simulink model "Inverse_model"  (R2021a)
settings: Solver=VariableStepAuto  StartTime=0.0  StopTime=1400  RelTol=1e-3
values from neighbouring files (symbols this model uses):
  B = 0.029    [project.m]
  J = 0.1    [project.m]
  ke = 0.6    [project.m]
  kt = 0.6    [project.m]
  La = 1e-3    (= 0.001)    [project.m]
  Ra = 1    [project.m]
libraries: pid_lib x6
settings Model: SimulationMode=rapid-accelerator  Creator=User  LastModifiedBy=User

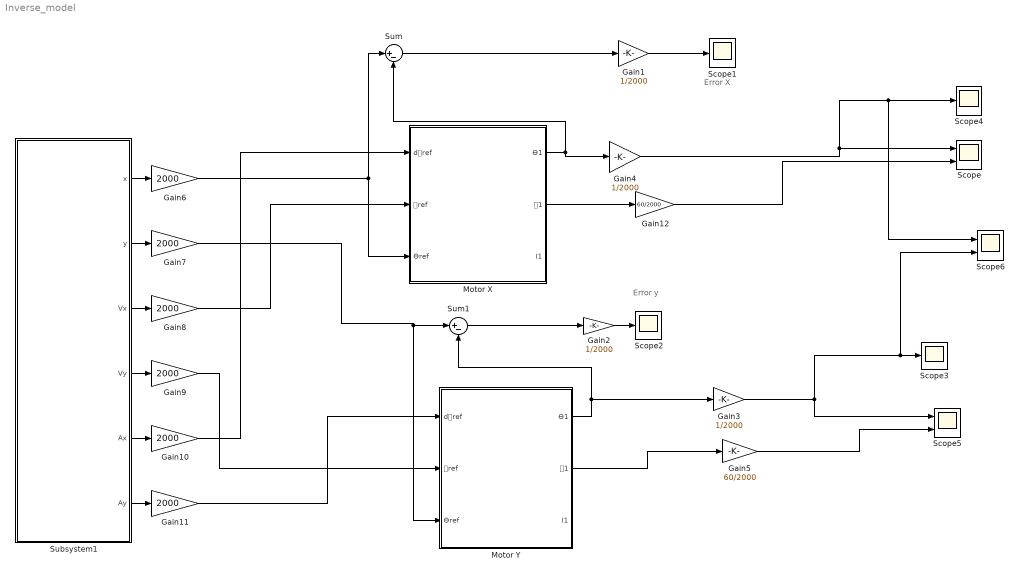
== system Inverse_model ==
  note: Error y
  note: Error X
  Gain{1..4} (4 alike) : Gain  Gain=1/2000
  Gain{6..11} (6 alike) : Gain  Gain=2000
  Gain12 : Gain  Gain=60/2000
  Gain5 : Gain  Gain=60/2000
  Motor X : Subsystem
  Motor Y : Subsystem
  Scope : Scope  NumInputPorts=2
  Scope{1..4} (4 alike) : Scope
  Scope5 : Scope  NumInputPorts=2
  Scope6 : Scope  NumInputPorts=2
  Subsystem1 : Subsystem
  Sum : Sum  Inputs=|+-
  Sum1 : Sum  Inputs=|+-
  wires:
  Subsystem1/1(x) -> Gain6/1
  Subsystem1/3(Vx) -> Gain8/1
  Subsystem1/5(Ax) -> Gain10/1
  Subsystem1/2(y) -> Gain7/1
  Subsystem1/4(Vy) -> Gain9/1
  Subsystem1/6(Ay) -> Gain11/1
  Sum1/1 -> Gain2/1
  Gain2/1 -> Scope2/1
  Gain3/1 -> Scope5/1, Scope6/2, Scope3/1
  Motor X/2(Ꞷ1) -> Gain12/1
  Gain6/1 -> Motor X/3(Ѳref), Sum/1
  Gain7/1 -> Sum1/1, Motor Y/3(Ѳref)
  Gain8/1 -> Motor X/2(Ꞷref)
  Gain10/1 -> Motor X/1(dꞶref)
  Gain9/1 -> Motor Y/2(Ꞷref)
  Gain11/1 -> Motor Y/1(dꞶref)
  Gain5/1 -> Scope5/2
  Motor X/1(Ѳ1) -> Gain4/1, Sum/2
  Gain4/1 -> Scope/1, Scope6/1, Scope4/1
  Sum/1 -> Gain1/1
  Gain1/1 -> Scope1/1
  Gain12/1 -> Scope/2
  Motor Y/1(Ѳ1) -> Gain3/1, Sum1/2
  Motor Y/2(Ꞷ1) -> Gain5/1

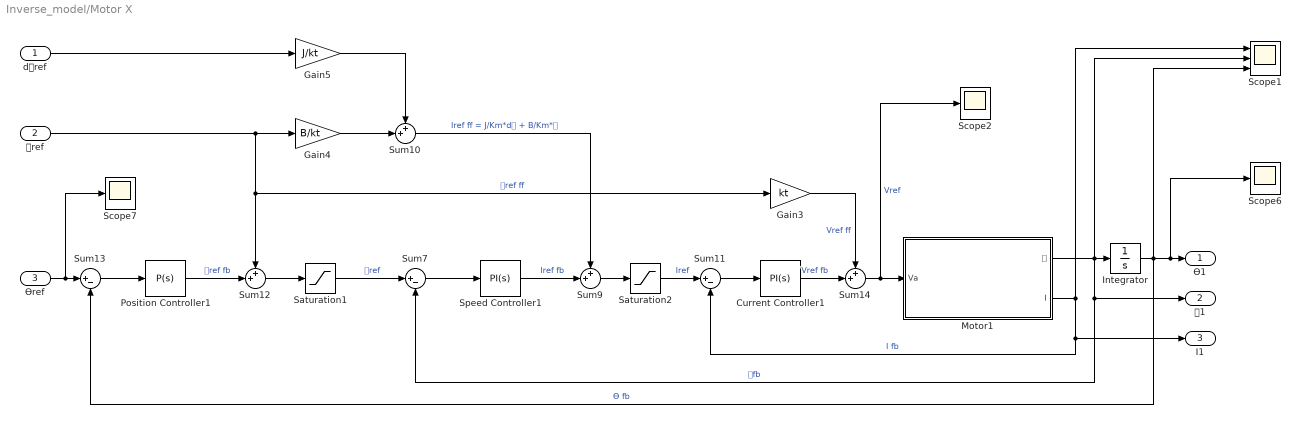
== system Inverse_model/Motor X ==
  dꞶref : Inport
  Ꞷref : Inport  Port=2
  Ѳref : Inport  Port=3
  Current Controller1 : pid_lib/PID Controller  Controller=PI  Form=Parallel  TimeDomain=Continuous-time  UseExternalTs=off  SampleTime=-1  IntegratorMethod=Forward Euler  FilterMethod=Forward Euler  ControllerParametersSource=internal  P=1000*La  I=1000*Ra  D=0  UseFilter=on  N=100  TunerSelectOption=Frequency Response Based  InitialConditionSource=internal  InitialConditionForIntegrator=0  InitialConditionForFilter=0  DifferentiatorICPrevScaledInput=0  ExternalReset=none  TrackingMode=off  Kt=1  LimitOutput=off  SatLimitsSource=internal  UpperSaturationLimit=inf  LowerSaturationLimit=-inf  LinearizeAsGain=on  AntiWindupMode=none  Kb=1  POutMin=[]  POutMax=[]  IOutMin=[]  IOutMax=[]  DOutMin=[]  DOutMax=[]  NOutMin=[]  NOutMax=[]  SumOutMin=[]  SumOutMax=[]  SaturationOutMin=[]  SaturationOutMax=[]  PParamMin=[]  PParamMax=[]  IParamMin=[]  IParamMax=[]  DParamMin=[]  DParamMax=[]  NParamMin=[]  NParamMax=[]  KbParamMin=[]  KbParamMax=[]  KtParamMin=[]  KtParamMax=[]  KbOutMin=[]  KbOutMax=[]  KtOutMin=[]  KtOutMax=[]  IntegratorOutMin=[]  IntegratorOutMax=[]  FilterOutMin=[]  FilterOutMax=[]  SumI1OutMin=[]  SumI1OutMax=[]  SumI2OutMin=[]  SumI2OutMax=[]  SumI3OutMin=[]  SumI3OutMax=[]  SumI4OutMin=[]  SumI4OutMax=[]  SumDOutMin=[]  SumDOutMax=[]  DifferentiatorOutMin=[]  DifferentiatorOutMax=[]  FilterDiffOutCoefMin=[]  FilterDiffOutCoefMax=[]  ReciprocalOutMin=[]  ReciprocalOutMax=[]  SumDenOutMin=[]  SumDenOutMax=[]  SumNumOutMin=[]  SumNumOutMax=[]  DivideOutMin=[]  DivideOutMax=[]  UdiffTsProdOutMin=[]  UdiffTsProdOutMax=[]  NTsProdOutMin=[]  NTsProdOutMax=[]  UintegralTsProdOutMin=[]  UintegralTsProdOutMax=[]  UngainTsProdOutMin=[]  UngainTsProdOutMax=[]  IntegratorContinuousStateAttributes=''  IntegratorStateMustResolveToSignalObject=off  IntegratorRTWStateStorageClass=Auto  FilterContinuousStateAttributes=''  FilterStateMustResolveToSignalObject=off  FilterRTWStateStorageClass=Auto  ParallelPVariant=InternalParameters  IdealPVariant=Disabled  IVariant=InternalParameters  DVariant=Disabled  IntegratorVariant=Continuous  SatVariant=Disabled  AWVariant=Passthrough  PCopyVariant=Disabled  TRVariant=Disabled  FdbkBlocksVariant=Forward  IdealPFdbkVariant=Disabled  SatFdbkVariant=Disabled  DerivativeFilterVariant=Disabled  NVariant=Disabled  NCopyVariant=Disabled_SignalSpec  FilterICVariant=Disabled  IntegratorICVariant=InternalICs  ExternalResetVariant=Disabled  TRSumVariant=Passthrough  SumFdbkVariant=Disabled  SumVariant=Sum_PI  TsampFilterVariant=InternalTs  TsampNgainVariant=Passthrough  TsampIntegralVariant=Passthrough  ExternalSaturationOutDataTypeStr=Inherit: Same as second input
  Gain3 : Gain  Gain=kt
  Gain4 : Gain  Gain=B/kt
  Gain5 : Gain  Gain=J/kt
  Integrator : Integrator  InitialCondition=6000
  Motor1 : Subsystem
  Position Controller1 : pid_lib/PID Controller  Controller=P  Form=Parallel  TimeDomain=Continuous-time  UseExternalTs=off  SampleTime=-1  IntegratorMethod=Forward Euler  FilterMethod=Forward Euler  ControllerParametersSource=internal  P=10  I=1  D=0  UseFilter=on  N=100  TunerSelectOption=Frequency Response Based  InitialConditionSource=internal  InitialConditionForIntegrator=0  InitialConditionForFilter=0  DifferentiatorICPrevScaledInput=0  ExternalReset=none  TrackingMode=off  Kt=1  LimitOutput=off  SatLimitsSource=internal  UpperSaturationLimit=inf  LowerSaturationLimit=-inf  LinearizeAsGain=on  AntiWindupMode=none  Kb=1  POutMin=[]  POutMax=[]  IOutMin=[]  IOutMax=[]  DOutMin=[]  DOutMax=[]  NOutMin=[]  NOutMax=[]  SumOutMin=[]  SumOutMax=[]  SaturationOutMin=[]  SaturationOutMax=[]  PParamMin=[]  PParamMax=[]  IParamMin=[]  IParamMax=[]  DParamMin=[]  DParamMax=[]  NParamMin=[]  NParamMax=[]  KbParamMin=[]  KbParamMax=[]  KtParamMin=[]  KtParamMax=[]  KbOutMin=[]  KbOutMax=[]  KtOutMin=[]  KtOutMax=[]  IntegratorOutMin=[]  IntegratorOutMax=[]  FilterOutMin=[]  FilterOutMax=[]  SumI1OutMin=[]  SumI1OutMax=[]  SumI2OutMin=[]  SumI2OutMax=[]  SumI3OutMin=[]  SumI3OutMax=[]  SumI4OutMin=[]  SumI4OutMax=[]  SumDOutMin=[]  SumDOutMax=[]  DifferentiatorOutMin=[]  DifferentiatorOutMax=[]  FilterDiffOutCoefMin=[]  FilterDiffOutCoefMax=[]  ReciprocalOutMin=[]  ReciprocalOutMax=[]  SumDenOutMin=[]  SumDenOutMax=[]  SumNumOutMin=[]  SumNumOutMax=[]  DivideOutMin=[]  DivideOutMax=[]  UdiffTsProdOutMin=[]  UdiffTsProdOutMax=[]  NTsProdOutMin=[]  NTsProdOutMax=[]  UintegralTsProdOutMin=[]  UintegralTsProdOutMax=[]  UngainTsProdOutMin=[]  UngainTsProdOutMax=[]  IntegratorContinuousStateAttributes=''  IntegratorStateMustResolveToSignalObject=off  IntegratorRTWStateStorageClass=Auto  FilterContinuousStateAttributes=''  FilterStateMustResolveToSignalObject=off  FilterRTWStateStorageClass=Auto  ParallelPVariant=InternalParameters  IdealPVariant=Disabled  IVariant=Disabled  DVariant=Disabled  IntegratorVariant=Disabled  SatVariant=Disabled  AWVariant=Disabled  PCopyVariant=Disabled  TRVariant=Disabled  FdbkBlocksVariant=Forward  IdealPFdbkVariant=Disabled  SatFdbkVariant=Disabled  DerivativeFilterVariant=Disabled  NVariant=Disabled  NCopyVariant=Disabled_SignalSpec  FilterICVariant=Disabled  IntegratorICVariant=Disabled  ExternalResetVariant=Disabled  TRSumVariant=Passthrough  SumFdbkVariant=Disabled  SumVariant=Passthrough_P  TsampFilterVariant=InternalTs  TsampNgainVariant=Passthrough  TsampIntegralVariant=Disabled_SignalSpec  ExternalSaturationOutDataTypeStr=Inherit: Same as second input
  Saturation1 : Saturate  UpperLimit=3000  LowerLimit=-3000
  Saturation2 : Saturate  UpperLimit=3000  LowerLimit=-3000
  Scope1 : Scope  NumInputPorts=3
  Scope2 : Scope
  Scope6 : Scope
  Scope7 : Scope
  Speed Controller1 : pid_lib/PID Controller  Controller=PI  Form=Parallel  TimeDomain=Continuous-time  UseExternalTs=off  SampleTime=-1  IntegratorMethod=Forward Euler  FilterMethod=Forward Euler  ControllerParametersSource=internal  P=344*J  I=344*B  D=2.5  UseFilter=on  N=100  TunerSelectOption=Transfer Function Based (PID Tuner App)  InitialConditionSource=internal  InitialConditionForIntegrator=0  InitialConditionForFilter=0  DifferentiatorICPrevScaledInput=0  ExternalReset=none  TrackingMode=off  Kt=1  LimitOutput=off  SatLimitsSource=internal  UpperSaturationLimit=inf  LowerSaturationLimit=-inf  LinearizeAsGain=on  AntiWindupMode=none  Kb=1  POutMin=[]  POutMax=[]  IOutMin=[]  IOutMax=[]  DOutMin=[]  DOutMax=[]  NOutMin=[]  NOutMax=[]  SumOutMin=[]  SumOutMax=[]  SaturationOutMin=[]  SaturationOutMax=[]  PParamMin=[]  PParamMax=[]  IParamMin=[]  IParamMax=[]  DParamMin=[]  DParamMax=[]  NParamMin=[]  NParamMax=[]  KbParamMin=[]  KbParamMax=[]  KtParamMin=[]  KtParamMax=[]  KbOutMin=[]  KbOutMax=[]  KtOutMin=[]  KtOutMax=[]  IntegratorOutMin=[]  IntegratorOutMax=[]  FilterOutMin=[]  FilterOutMax=[]  SumI1OutMin=[]  SumI1OutMax=[]  SumI2OutMin=[]  SumI2OutMax=[]  SumI3OutMin=[]  SumI3OutMax=[]  SumI4OutMin=[]  SumI4OutMax=[]  SumDOutMin=[]  SumDOutMax=[]  DifferentiatorOutMin=[]  DifferentiatorOutMax=[]  FilterDiffOutCoefMin=[]  FilterDiffOutCoefMax=[]  ReciprocalOutMin=[]  ReciprocalOutMax=[]  SumDenOutMin=[]  SumDenOutMax=[]  SumNumOutMin=[]  SumNumOutMax=[]  DivideOutMin=[]  DivideOutMax=[]  UdiffTsProdOutMin=[]  UdiffTsProdOutMax=[]  NTsProdOutMin=[]  NTsProdOutMax=[]  UintegralTsProdOutMin=[]  UintegralTsProdOutMax=[]  UngainTsProdOutMin=[]  UngainTsProdOutMax=[]  IntegratorContinuousStateAttributes=''  IntegratorStateMustResolveToSignalObject=off  IntegratorRTWStateStorageClass=Auto  FilterContinuousStateAttributes=''  FilterStateMustResolveToSignalObject=off  FilterRTWStateStorageClass=Auto  ParallelPVariant=InternalParameters  IdealPVariant=Disabled  IVariant=InternalParameters  DVariant=Disabled  IntegratorVariant=Continuous  SatVariant=Disabled  AWVariant=Passthrough  PCopyVariant=Disabled  TRVariant=Disabled  FdbkBlocksVariant=Forward  IdealPFdbkVariant=Disabled  SatFdbkVariant=Disabled  DerivativeFilterVariant=Disabled  NVariant=Disabled  NCopyVariant=Disabled_SignalSpec  FilterICVariant=Disabled  IntegratorICVariant=InternalICs  ExternalResetVariant=Disabled  TRSumVariant=Passthrough  SumFdbkVariant=Disabled  SumVariant=Sum_PI  TsampFilterVariant=InternalTs  TsampNgainVariant=Passthrough  TsampIntegralVariant=Passthrough  ExternalSaturationOutDataTypeStr=Inherit: Same as second input
  Sum{9..10,12,14} (4 alike) : Sum  Inputs=++|
  Sum11 : Sum  Inputs=|+-
  Sum13 : Sum  Inputs=|+-
  Sum7 : Sum  Inputs=|+-
  Ѳ1 : Outport  VectorParamsAs1DForOutWhenUnconnected=off
  Ꞷ1 : Outport  Port=2  VectorParamsAs1DForOutWhenUnconnected=off
  I1 : Outport  Port=3  VectorParamsAs1DForOutWhenUnconnected=off
  wires:
  Current Controller1/1 -> Sum14/2  "Vref fb"
  Sum10/1 -> Sum9/1  "Iref ff = J/Km*dꞶ + B/Km*Ꞷ"
  Gain3/1 -> Sum14/1  "Vref ff"
  Motor1/1(Ꞷ) -> Scope1/2, Integrator/1, Sum7/2, Ꞷ1/1  "Ꞷfb"
  Saturation2/1 -> Sum11/1  "Iref"
  Integrator/1 -> Scope1/3, Scope6/1, Ѳ1/1, Sum13/2  "Ѳ fb"
  Speed Controller1/1 -> Sum9/2  "Iref fb"
  Gain4/1 -> Sum10/2
  Position Controller1/1 -> Sum12/2  "Ꞷref fb"
  Ꞷref/1 -> Gain3/1, Sum12/1, Gain4/1  "Ꞷref ff"
  Motor1/2(I) -> Scope1/1, I1/1, Sum11/2  "I fb"
  dꞶref/1 -> Gain5/1
  Ѳref/1 -> Scope7/1, Sum13/1
  Sum12/1 -> Saturation1/1
  Gain5/1 -> Sum10/1
  Sum11/1 -> Current Controller1/1
  Sum7/1 -> Speed Controller1/1
  Sum14/1 -> Scope2/1, Motor1/1(Va)  "Vref"
  Sum9/1 -> Saturation2/1
  Sum13/1 -> Position Controller1/1
  Saturation1/1 -> Sum7/1  "Ꞷref"

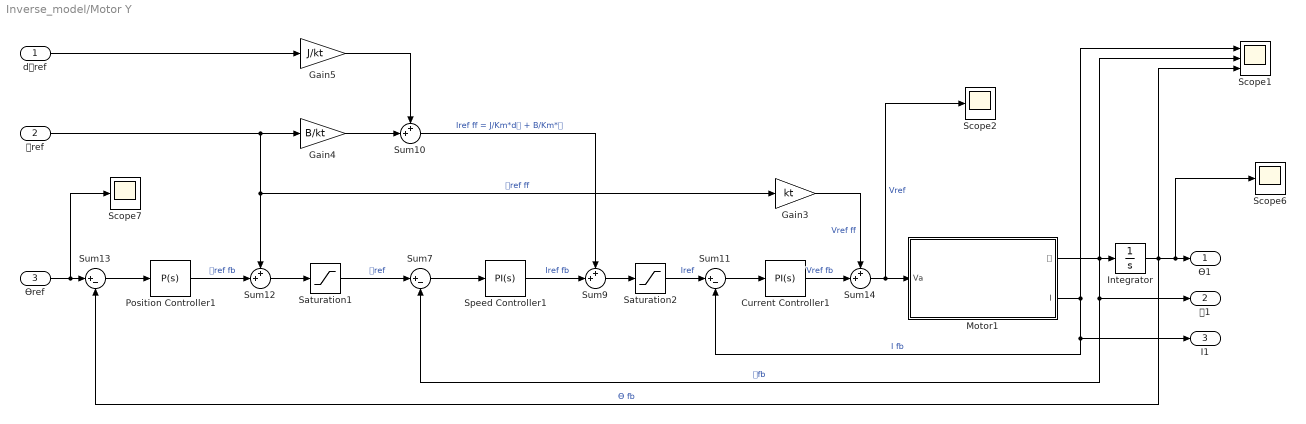
== system Inverse_model/Motor Y ==
  dꞶref : Inport
  Ꞷref : Inport  Port=2
  Ѳref : Inport  Port=3
  Current Controller1 : pid_lib/PID Controller  Controller=PI  Form=Parallel  TimeDomain=Continuous-time  UseExternalTs=off  SampleTime=-1  IntegratorMethod=Forward Euler  FilterMethod=Forward Euler  ControllerParametersSource=internal  P=1000*La  I=1000*Ra  D=0  UseFilter=on  N=100  TunerSelectOption=Frequency Response Based  InitialConditionSource=internal  InitialConditionForIntegrator=0  InitialConditionForFilter=0  DifferentiatorICPrevScaledInput=0  ExternalReset=none  TrackingMode=off  Kt=1  LimitOutput=off  SatLimitsSource=internal  UpperSaturationLimit=inf  LowerSaturationLimit=-inf  LinearizeAsGain=on  AntiWindupMode=none  Kb=1  POutMin=[]  POutMax=[]  IOutMin=[]  IOutMax=[]  DOutMin=[]  DOutMax=[]  NOutMin=[]  NOutMax=[]  SumOutMin=[]  SumOutMax=[]  SaturationOutMin=[]  SaturationOutMax=[]  PParamMin=[]  PParamMax=[]  IParamMin=[]  IParamMax=[]  DParamMin=[]  DParamMax=[]  NParamMin=[]  NParamMax=[]  KbParamMin=[]  KbParamMax=[]  KtParamMin=[]  KtParamMax=[]  KbOutMin=[]  KbOutMax=[]  KtOutMin=[]  KtOutMax=[]  IntegratorOutMin=[]  IntegratorOutMax=[]  FilterOutMin=[]  FilterOutMax=[]  SumI1OutMin=[]  SumI1OutMax=[]  SumI2OutMin=[]  SumI2OutMax=[]  SumI3OutMin=[]  SumI3OutMax=[]  SumI4OutMin=[]  SumI4OutMax=[]  SumDOutMin=[]  SumDOutMax=[]  DifferentiatorOutMin=[]  DifferentiatorOutMax=[]  FilterDiffOutCoefMin=[]  FilterDiffOutCoefMax=[]  ReciprocalOutMin=[]  ReciprocalOutMax=[]  SumDenOutMin=[]  SumDenOutMax=[]  SumNumOutMin=[]  SumNumOutMax=[]  DivideOutMin=[]  DivideOutMax=[]  UdiffTsProdOutMin=[]  UdiffTsProdOutMax=[]  NTsProdOutMin=[]  NTsProdOutMax=[]  UintegralTsProdOutMin=[]  UintegralTsProdOutMax=[]  UngainTsProdOutMin=[]  UngainTsProdOutMax=[]  IntegratorContinuousStateAttributes=''  IntegratorStateMustResolveToSignalObject=off  IntegratorRTWStateStorageClass=Auto  FilterContinuousStateAttributes=''  FilterStateMustResolveToSignalObject=off  FilterRTWStateStorageClass=Auto  ParallelPVariant=InternalParameters  IdealPVariant=Disabled  IVariant=InternalParameters  DVariant=Disabled  IntegratorVariant=Continuous  SatVariant=Disabled  AWVariant=Passthrough  PCopyVariant=Disabled  TRVariant=Disabled  FdbkBlocksVariant=Forward  IdealPFdbkVariant=Disabled  SatFdbkVariant=Disabled  DerivativeFilterVariant=Disabled  NVariant=Disabled  NCopyVariant=Disabled_SignalSpec  FilterICVariant=Disabled  IntegratorICVariant=InternalICs  ExternalResetVariant=Disabled  TRSumVariant=Passthrough  SumFdbkVariant=Disabled  SumVariant=Sum_PI  TsampFilterVariant=InternalTs  TsampNgainVariant=Passthrough  TsampIntegralVariant=Passthrough  ExternalSaturationOutDataTypeStr=Inherit: Same as second input
  Gain3 : Gain  Gain=kt
  Gain4 : Gain  Gain=B/kt
  Gain5 : Gain  Gain=J/kt
  Integrator : Integrator  InitialCondition=4000
  Motor1 : Subsystem
  Position Controller1 : pid_lib/PID Controller  Controller=P  Form=Parallel  TimeDomain=Continuous-time  UseExternalTs=off  SampleTime=-1  IntegratorMethod=Forward Euler  FilterMethod=Forward Euler  ControllerParametersSource=internal  P=10  I=1  D=0  UseFilter=on  N=100  TunerSelectOption=Frequency Response Based  InitialConditionSource=internal  InitialConditionForIntegrator=0  InitialConditionForFilter=0  DifferentiatorICPrevScaledInput=0  ExternalReset=none  TrackingMode=off  Kt=1  LimitOutput=off  SatLimitsSource=internal  UpperSaturationLimit=inf  LowerSaturationLimit=-inf  LinearizeAsGain=on  AntiWindupMode=none  Kb=1  POutMin=[]  POutMax=[]  IOutMin=[]  IOutMax=[]  DOutMin=[]  DOutMax=[]  NOutMin=[]  NOutMax=[]  SumOutMin=[]  SumOutMax=[]  SaturationOutMin=[]  SaturationOutMax=[]  PParamMin=[]  PParamMax=[]  IParamMin=[]  IParamMax=[]  DParamMin=[]  DParamMax=[]  NParamMin=[]  NParamMax=[]  KbParamMin=[]  KbParamMax=[]  KtParamMin=[]  KtParamMax=[]  KbOutMin=[]  KbOutMax=[]  KtOutMin=[]  KtOutMax=[]  IntegratorOutMin=[]  IntegratorOutMax=[]  FilterOutMin=[]  FilterOutMax=[]  SumI1OutMin=[]  SumI1OutMax=[]  SumI2OutMin=[]  SumI2OutMax=[]  SumI3OutMin=[]  SumI3OutMax=[]  SumI4OutMin=[]  SumI4OutMax=[]  SumDOutMin=[]  SumDOutMax=[]  DifferentiatorOutMin=[]  DifferentiatorOutMax=[]  FilterDiffOutCoefMin=[]  FilterDiffOutCoefMax=[]  ReciprocalOutMin=[]  ReciprocalOutMax=[]  SumDenOutMin=[]  SumDenOutMax=[]  SumNumOutMin=[]  SumNumOutMax=[]  DivideOutMin=[]  DivideOutMax=[]  UdiffTsProdOutMin=[]  UdiffTsProdOutMax=[]  NTsProdOutMin=[]  NTsProdOutMax=[]  UintegralTsProdOutMin=[]  UintegralTsProdOutMax=[]  UngainTsProdOutMin=[]  UngainTsProdOutMax=[]  IntegratorContinuousStateAttributes=''  IntegratorStateMustResolveToSignalObject=off  IntegratorRTWStateStorageClass=Auto  FilterContinuousStateAttributes=''  FilterStateMustResolveToSignalObject=off  FilterRTWStateStorageClass=Auto  ParallelPVariant=InternalParameters  IdealPVariant=Disabled  IVariant=Disabled  DVariant=Disabled  IntegratorVariant=Disabled  SatVariant=Disabled  AWVariant=Disabled  PCopyVariant=Disabled  TRVariant=Disabled  FdbkBlocksVariant=Forward  IdealPFdbkVariant=Disabled  SatFdbkVariant=Disabled  DerivativeFilterVariant=Disabled  NVariant=Disabled  NCopyVariant=Disabled_SignalSpec  FilterICVariant=Disabled  IntegratorICVariant=Disabled  ExternalResetVariant=Disabled  TRSumVariant=Passthrough  SumFdbkVariant=Disabled  SumVariant=Passthrough_P  TsampFilterVariant=InternalTs  TsampNgainVariant=Passthrough  TsampIntegralVariant=Disabled_SignalSpec  ExternalSaturationOutDataTypeStr=Inherit: Same as second input
  Saturation1 : Saturate  UpperLimit=3000  LowerLimit=-3000
  Saturation2 : Saturate  UpperLimit=3000  LowerLimit=-3000
  Scope1 : Scope  NumInputPorts=3
  Scope2 : Scope
  Scope6 : Scope
  Scope7 : Scope
  Speed Controller1 : pid_lib/PID Controller  Controller=PI  Form=Parallel  TimeDomain=Continuous-time  UseExternalTs=off  SampleTime=-1  IntegratorMethod=Forward Euler  FilterMethod=Forward Euler  ControllerParametersSource=internal  P=344*J  I=344*B  D=2.5  UseFilter=on  N=100  TunerSelectOption=Transfer Function Based (PID Tuner App)  InitialConditionSource=internal  InitialConditionForIntegrator=0  InitialConditionForFilter=0  DifferentiatorICPrevScaledInput=0  ExternalReset=none  TrackingMode=off  Kt=1  LimitOutput=off  SatLimitsSource=internal  UpperSaturationLimit=inf  LowerSaturationLimit=-inf  LinearizeAsGain=on  AntiWindupMode=none  Kb=1  POutMin=[]  POutMax=[]  IOutMin=[]  IOutMax=[]  DOutMin=[]  DOutMax=[]  NOutMin=[]  NOutMax=[]  SumOutMin=[]  SumOutMax=[]  SaturationOutMin=[]  SaturationOutMax=[]  PParamMin=[]  PParamMax=[]  IParamMin=[]  IParamMax=[]  DParamMin=[]  DParamMax=[]  NParamMin=[]  NParamMax=[]  KbParamMin=[]  KbParamMax=[]  KtParamMin=[]  KtParamMax=[]  KbOutMin=[]  KbOutMax=[]  KtOutMin=[]  KtOutMax=[]  IntegratorOutMin=[]  IntegratorOutMax=[]  FilterOutMin=[]  FilterOutMax=[]  SumI1OutMin=[]  SumI1OutMax=[]  SumI2OutMin=[]  SumI2OutMax=[]  SumI3OutMin=[]  SumI3OutMax=[]  SumI4OutMin=[]  SumI4OutMax=[]  SumDOutMin=[]  SumDOutMax=[]  DifferentiatorOutMin=[]  DifferentiatorOutMax=[]  FilterDiffOutCoefMin=[]  FilterDiffOutCoefMax=[]  ReciprocalOutMin=[]  ReciprocalOutMax=[]  SumDenOutMin=[]  SumDenOutMax=[]  SumNumOutMin=[]  SumNumOutMax=[]  DivideOutMin=[]  DivideOutMax=[]  UdiffTsProdOutMin=[]  UdiffTsProdOutMax=[]  NTsProdOutMin=[]  NTsProdOutMax=[]  UintegralTsProdOutMin=[]  UintegralTsProdOutMax=[]  UngainTsProdOutMin=[]  UngainTsProdOutMax=[]  IntegratorContinuousStateAttributes=''  IntegratorStateMustResolveToSignalObject=off  IntegratorRTWStateStorageClass=Auto  FilterContinuousStateAttributes=''  FilterStateMustResolveToSignalObject=off  FilterRTWStateStorageClass=Auto  ParallelPVariant=InternalParameters  IdealPVariant=Disabled  IVariant=InternalParameters  DVariant=Disabled  IntegratorVariant=Continuous  SatVariant=Disabled  AWVariant=Passthrough  PCopyVariant=Disabled  TRVariant=Disabled  FdbkBlocksVariant=Forward  IdealPFdbkVariant=Disabled  SatFdbkVariant=Disabled  DerivativeFilterVariant=Disabled  NVariant=Disabled  NCopyVariant=Disabled_SignalSpec  FilterICVariant=Disabled  IntegratorICVariant=InternalICs  ExternalResetVariant=Disabled  TRSumVariant=Passthrough  SumFdbkVariant=Disabled  SumVariant=Sum_PI  TsampFilterVariant=InternalTs  TsampNgainVariant=Passthrough  TsampIntegralVariant=Passthrough  ExternalSaturationOutDataTypeStr=Inherit: Same as second input
  Sum{9..10,12,14} (4 alike) : Sum  Inputs=++|
  Sum11 : Sum  Inputs=|+-
  Sum13 : Sum  Inputs=|+-
  Sum7 : Sum  Inputs=|+-
  Ѳ1 : Outport  VectorParamsAs1DForOutWhenUnconnected=off
  Ꞷ1 : Outport  Port=2  VectorParamsAs1DForOutWhenUnconnected=off
  I1 : Outport  Port=3  VectorParamsAs1DForOutWhenUnconnected=off
  wires:
  Saturation1/1 -> Sum7/1  "Ꞷref"
  Sum13/1 -> Position Controller1/1
  Sum11/1 -> Current Controller1/1
  Gain5/1 -> Sum10/1
  Sum12/1 -> Saturation1/1
  Gain4/1 -> Sum10/2
  Speed Controller1/1 -> Sum9/2  "Iref fb"
  Position Controller1/1 -> Sum12/2  "Ꞷref fb"
  Sum9/1 -> Saturation2/1
  Saturation2/1 -> Sum11/1  "Iref"
  Gain3/1 -> Sum14/1  "Vref ff"
  Motor1/1(Ꞷ) -> Scope1/2, Integrator/1, Sum7/2, Ꞷ1/1  "Ꞷfb"
  Sum14/1 -> Scope2/1, Motor1/1(Va)  "Vref"
  Current Controller1/1 -> Sum14/2  "Vref fb"
  Sum7/1 -> Speed Controller1/1
  Sum10/1 -> Sum9/1  "Iref ff = J/Km*dꞶ + B/Km*Ꞷ"
  Integrator/1 -> Scope1/3, Scope6/1, Ѳ1/1, Sum13/2  "Ѳ fb"
  Ꞷref/1 -> Gain3/1, Sum12/1, Gain4/1  "Ꞷref ff"
  dꞶref/1 -> Gain5/1
  Ѳref/1 -> Scope7/1, Sum13/1
  Motor1/2(I) -> Scope1/1, I1/1, Sum11/2  "I fb"

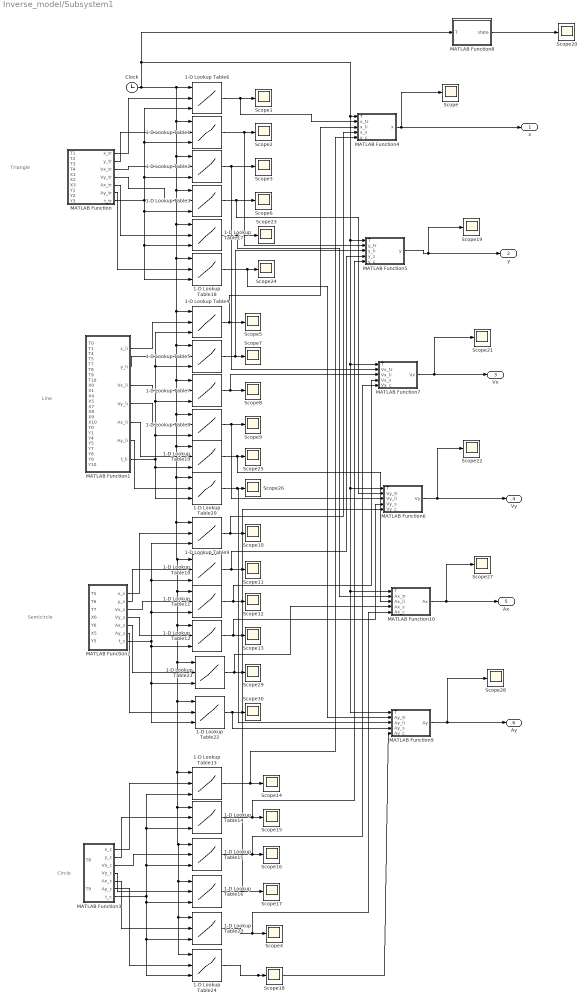
== system Inverse_model/Subsystem1 ==
  note: Circle
  note: Semicircle
  note: Line
  note: Triangle
  1-D Lookup Table{1..24} (24 alike) : Lookup_n-D  NumberOfTableDimensions=1  BreakpointsForDimension1Source=Input port  BreakpointsForDimension1=[-5:5]  TableSource=Input port  Table=tanh([-5:5])  InternalRulePriority=Speed  RndMeth=Simplest  InputSameDT=on
      settings: InputPortMap=u0,p221,p5
  Clock : Clock
  MATLAB Function : MATLAB Function  TreatAsAtomicUnit=on
  MATLAB Function1 : MATLAB Function  TreatAsAtomicUnit=on
  MATLAB Function10 : MATLAB Function  TreatAsAtomicUnit=on
  MATLAB Function2 : MATLAB Function  TreatAsAtomicUnit=on
  MATLAB Function3 : MATLAB Function  TreatAsAtomicUnit=on
  MATLAB Function4 : MATLAB Function  TreatAsAtomicUnit=on
  MATLAB Function5 : MATLAB Function  TreatAsAtomicUnit=on
  MATLAB Function6 : MATLAB Function  TreatAsAtomicUnit=on
  MATLAB Function7 : MATLAB Function  TreatAsAtomicUnit=on
  MATLAB Function8 : MATLAB Function  TreatAsAtomicUnit=on
  MATLAB Function9 : MATLAB Function  TreatAsAtomicUnit=on
  Scope{,1..30} (31 alike) : Scope
  x : Outport
  y : Outport  Port=2
  Vx : Outport  Port=3
  Vy : Outport  Port=4
  Ax : Outport  Port=5
  Ay : Outport  Port=6
  wires:
  Clock/1 -> 1-D Lookup Table24/1, 1-D Lookup Table23/1, 1-D Lookup Table16/1, 1-D Lookup Table15/1, 1-D Lookup Table14/1, 1-D Lookup Table13/1, 1-D Lookup Table22/1, 1-D Lookup Table21/1, 1-D Lookup Table12/1, 1-D Lookup Table11/1, 1-D Lookup Table10/1, 1-D Lookup Table9/1, 1-D Lookup Table20/1, 1-D Lookup Table19/1, 1-D Lookup Table8/1, 1-D Lookup Table7/1, 1-D Lookup Table5/1, 1-D Lookup Table4/1, 1-D Lookup Table18/1, 1-D Lookup Table17/1, 1-D Lookup Table3/1, 1-D Lookup Table2/1, 1-D Lookup Table1/1, 1-D Lookup Table6/1, MATLAB Function9/1(T), MATLAB Function10/1(T), MATLAB Function6/1(T), MATLAB Function7/1(T), MATLAB Function5/1(T), MATLAB Function4/1(T), MATLAB Function8/1(T)
  1-D Lookup Table6/1 -> MATLAB Function4/2(x_tr), Scope1/1
  1-D Lookup Table1/1 -> MATLAB Function5/2(y_tr), Scope2/1
  1-D Lookup Table2/1 -> MATLAB Function7/2(Vx_tr), Scope3/1
  1-D Lookup Table4/1 -> MATLAB Function4/3(x_li), Scope5/1
  1-D Lookup Table7/1 -> MATLAB Function7/3(Vx_li), Scope8/1
  1-D Lookup Table8/1 -> MATLAB Function6/3(Vy_li), Scope9/1
  1-D Lookup Table9/1 -> MATLAB Function4/4(x_s), Scope10/1
  1-D Lookup Table10/1 -> MATLAB Function5/4(y_s), Scope11/1
  1-D Lookup Table11/1 -> MATLAB Function7/4(Vx_s), Scope12/1
  1-D Lookup Table12/1 -> MATLAB Function6/4(Vy_s), Scope13/1
  1-D Lookup Table13/1 -> MATLAB Function4/5(x_c), Scope14/1
  1-D Lookup Table15/1 -> MATLAB Function7/5(Vx_c), Scope16/1
  1-D Lookup Table16/1 -> MATLAB Function6/5(Vy_c), Scope17/1
  1-D Lookup Table14/1 -> MATLAB Function5/5(y_c), Scope15/1
  1-D Lookup Table5/1 -> MATLAB Function5/3(y_li), Scope7/1
  MATLAB Function8/1(state) -> Scope20/1
  1-D Lookup Table17/1 -> MATLAB Function10/2(Ax_tr), Scope23/1
  1-D Lookup Table3/1 -> MATLAB Function6/2(Vy_tr), Scope6/1
  1-D Lookup Table18/1 -> MATLAB Function9/2(Ay_tr), Scope24/1
  1-D Lookup Table20/1 -> MATLAB Function9/3(Ay_li), Scope26/1
  1-D Lookup Table19/1 -> MATLAB Function10/3(Ax_li), Scope25/1
  1-D Lookup Table24/1 -> MATLAB Function9/5(Ay_c), Scope18/1
  1-D Lookup Table23/1 -> MATLAB Function10/5(Ax_c), Scope4/1
  MATLAB Function4/1(x) -> x/1, Scope/1
  MATLAB Function5/1(y) -> y/1, Scope19/1
  MATLAB Function7/1(Vx) -> Vx/1, Scope21/1
  MATLAB Function6/1(Vy) -> Vy/1, Scope22/1
  MATLAB Function10/1(Ax) -> Ax/1, Scope27/1
  MATLAB Function9/1(Ay) -> Ay/1, Scope28/1
  1-D Lookup Table22/1 -> MATLAB Function9/4(Ay_s), Scope30/1
  1-D Lookup Table21/1 -> MATLAB Function10/4(Ax_s), Scope29/1
  MATLAB Function3/7(t_c) -> 1-D Lookup Table16/3, 1-D Lookup Table24/3, 1-D Lookup Table23/3, 1-D Lookup Table13/3, 1-D Lookup Table14/3, 1-D Lookup Table15/3
  MATLAB Function3/6(Ay_c) -> 1-D Lookup Table24/2
  MATLAB Function3/5(Ax_c) -> 1-D Lookup Table23/2
  MATLAB Function3/1(x_c) -> 1-D Lookup Table13/2
  MATLAB Function3/2(y_c) -> 1-D Lookup Table14/2
  MATLAB Function3/3(Vx_c) -> 1-D Lookup Table15/2
  MATLAB Function3/4(Vy_c) -> 1-D Lookup Table16/2
  MATLAB Function2/7(t_s) -> 1-D Lookup Table9/3, 1-D Lookup Table10/3, 1-D Lookup Table11/3, 1-D Lookup Table12/3, 1-D Lookup Table21/3, 1-D Lookup Table22/3
  MATLAB Function2/1(x_s) -> 1-D Lookup Table9/2
  MATLAB Function2/2(y_s) -> 1-D Lookup Table10/2
  MATLAB Function2/3(Vx_s) -> 1-D Lookup Table11/2
  MATLAB Function2/4(Vy_s) -> 1-D Lookup Table12/2
  MATLAB Function2/5(Ax_s) -> 1-D Lookup Table21/2
  MATLAB Function2/6(Ay_s) -> 1-D Lookup Table22/2
  MATLAB Function1/1(x_li) -> 1-D Lookup Table4/2
  MATLAB Function1/2(y_li) -> 1-D Lookup Table5/2
  MATLAB Function1/3(Vx_li) -> 1-D Lookup Table7/2
  MATLAB Function1/4(Vy_li) -> 1-D Lookup Table8/2
  MATLAB Function1/5(Ax_li) -> 1-D Lookup Table19/2
  MATLAB Function1/6(Ay_li) -> 1-D Lookup Table20/2
  MATLAB Function1/7(t_li) -> 1-D Lookup Table5/3, 1-D Lookup Table4/3, 1-D Lookup Table7/3, 1-D Lookup Table8/3, 1-D Lookup Table19/3, 1-D Lookup Table20/3
  MATLAB Function/7(t_tr) -> 1-D Lookup Table18/3, 1-D Lookup Table17/3, 1-D Lookup Table3/3, 1-D Lookup Table1/3, 1-D Lookup Table6/3, 1-D Lookup Table2/3
  MATLAB Function/1(x_tr) -> 1-D Lookup Table6/2
  MATLAB Function/2(y_tr) -> 1-D Lookup Table1/2
  MATLAB Function/3(Vx_tr) -> 1-D Lookup Table2/2
  MATLAB Function/4(Vy_tr) -> 1-D Lookup Table3/2
  MATLAB Function/5(Ax_tr) -> 1-D Lookup Table17/2
  MATLAB Function/6(Ay_tr) -> 1-D Lookup Table18/2

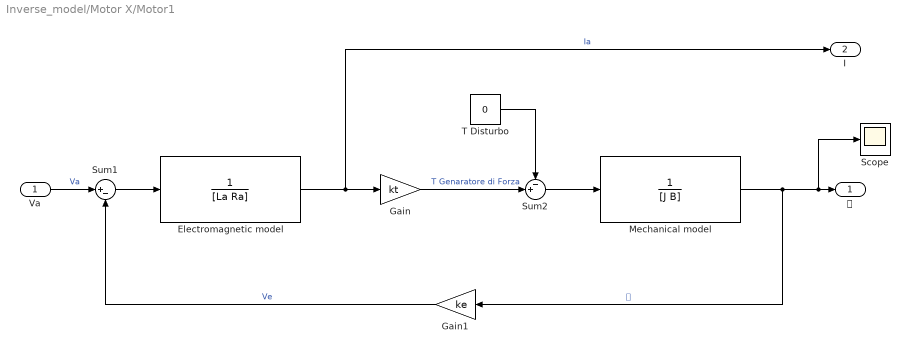
== system Inverse_model/Motor X/Motor1 ==
  Va : Inport
  Electromagnetic model : TransferFcn  Denominator=[La Ra]
  Gain : Gain  Gain=kt
  Gain1 : Gain  Gain=ke
  Mechanical model : TransferFcn  Denominator=[J B]
  Scope : Scope
  Sum1 : Sum  Inputs=|+-
  Sum2 : Sum  Inputs=-+|
  T Disturbo : Constant  Value=0
  Ꞷ : Outport  VectorParamsAs1DForOutWhenUnconnected=off
  I : Outport  Port=2  VectorParamsAs1DForOutWhenUnconnected=off
  wires:
  Va/1 -> Sum1/1  "Va"
  Sum1/1 -> Electromagnetic model/1
  Mechanical model/1 -> Gain1/1, Scope/1, Ꞷ/1  "Ꞷ"
  Electromagnetic model/1 -> Gain/1, I/1  "Ia"
  Gain1/1 -> Sum1/2  "Ve"
  Gain/1 -> Sum2/2  "T Genaratore di Forza"
  Sum2/1 -> Mechanical model/1
  T Disturbo/1 -> Sum2/1

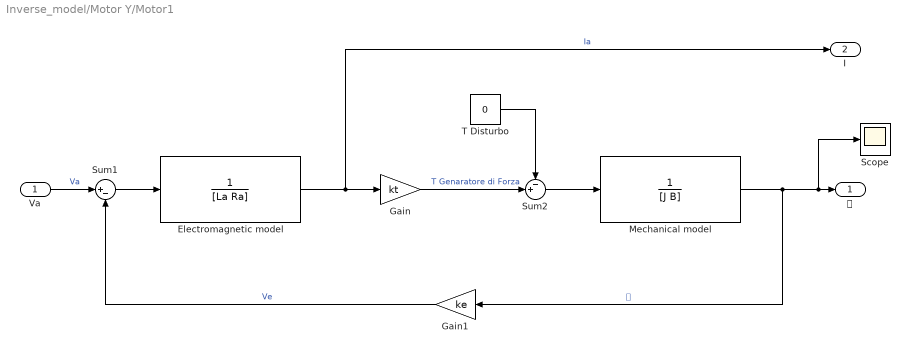
== system Inverse_model/Motor Y/Motor1 ==
  Va : Inport
  Electromagnetic model : TransferFcn  Denominator=[La Ra]
  Gain : Gain  Gain=kt
  Gain1 : Gain  Gain=ke
  Mechanical model : TransferFcn  Denominator=[J B]
  Scope : Scope
  Sum1 : Sum  Inputs=|+-
  Sum2 : Sum  Inputs=-+|
  T Disturbo : Constant  Value=0
  Ꞷ : Outport  VectorParamsAs1DForOutWhenUnconnected=off
  I : Outport  Port=2  VectorParamsAs1DForOutWhenUnconnected=off
  wires:
  Va/1 -> Sum1/1  "Va"
  Sum1/1 -> Electromagnetic model/1
  Mechanical model/1 -> Gain1/1, Scope/1, Ꞷ/1  "Ꞷ"
  Electromagnetic model/1 -> Gain/1, I/1  "Ia"
  Gain1/1 -> Sum1/2  "Ve"
  Gain/1 -> Sum2/2  "T Genaratore di Forza"
  Sum2/1 -> Mechanical model/1
  T Disturbo/1 -> Sum2/1

== matlab function Inverse_model/Subsystem1/MATLAB Function3 ==
  data: x_c output; T8 input; T9 input; y_c output; Vx_c output; Vy_c output; Ax_c output; Ay_c output; t_c output
function [x_c,y_c,Vx_c,Vy_c,Ax_c,Ay_c,t_c] = fcn(T8,T9)
T8=1005;
T9=1285;
t=T8:0.1:T9;
sigma=(t-T8)/(T9-T8);
lambda=poly5(sigma);
theta=lambda*2*pi;
R=0.5;
P=R*[cos(theta);sin(theta)];
x8=P(1,:)+2.25;
y8=P(2,:)+1;
lambdavel=poly5d(sigma);
Vx8=2*R*pi/(T9-T8)*lambdavel.*[-sin(theta)];
Vy8=2*R*pi/(T9-T8)*lambdavel.*[cos(theta)];
lambdaac=poly5dd(sigma);
Ax8=2*R*pi/(T9-T8)^2*lambdaac.*[-sin(theta)];
Ay8=2*R*pi/(T9-T8)^2*lambdaac.*[cos(theta)];
x_c=x8;
y_c=y8;
t_c=T8+sigma*(T9-T8);
Vx_c=Vx8;
Vy_c=Vy8;
Ax_c=Ax8;
Ay_c=Ay8;

== matlab function Inverse_model/Subsystem1/MATLAB Function4 ==
  data: T input; x output; x_tr input; x_li input; x_s input; x_c input
function x = fcn(T,x_tr,x_li,x_s,x_c)
if T>=260 && T<=530
    x=x_tr
elseif T>=675 && T<=905
    x=x_s
elseif T>=1005 && T<=1285
    x=x_c
else
    x=x_li
end

== matlab function Inverse_model/Subsystem1/MATLAB Function5 ==
  data: T input; y output; y_tr input; y_li input; y_s input; y_c input
function y = fcn(T,y_tr,y_li,y_s,y_c)
if T>=260 && T<=530
    y=y_tr
elseif T>=675 && T<=905
    y=y_s
elseif T>=1005 && T<=1285
    y=y_c
else
    y=y_li
end

== matlab function Inverse_model/Subsystem1/MATLAB Function6 ==
  data: T input; Vy output; Vy_tr input; Vy_li input; Vy_s input; Vy_c input
function Vy = fcn(T,Vy_tr,Vy_li,Vy_s,Vy_c)
if T>=260 && T<=530
    Vy=Vy_tr
elseif T>=675 && T<=905
    Vy=Vy_s
elseif T>=1005 && T<=1285
    Vy=Vy_c
else
    Vy=Vy_li
end

== matlab function Inverse_model/Subsystem1/MATLAB Function7 ==
  data: T input; Vx output; Vx_tr input; Vx_li input; Vx_s input; Vx_c input
function Vx = fcn(T,Vx_tr,Vx_li,Vx_s,Vx_c)
if T>=260 && T<=530
    Vx=Vx_tr
elseif T>=675 && T<=905
    Vx=Vx_s
elseif T>=1005 && T<=1285
    Vx=Vx_c
else
    Vx=Vx_li
end

== matlab function Inverse_model/Subsystem1/MATLAB Function8 ==
  data: T input; state output
function state = fcn(T)
if T>=260 && T<=530
    state=true
elseif T>=675 && T<=905
    state=true
elseif T>=1005 && T<=1285
    state=true
else
    state=false
end

== matlab function Inverse_model/Subsystem1/MATLAB Function9 ==
  data: T input; Ay output; Ay_tr input; Ay_li input; Ay_s input; Ay_c input
function Ay = fcn(T,Ay_tr,Ay_li,Ay_s,Ay_c)
if T>=260 && T<=530
    Ay=Ay_tr
elseif T>=675 && T<=905
    Ay=Ay_s
elseif T>=1005 && T<=1285
    Ay=Ay_c
else
    Ay=Ay_li
end

== matlab function Inverse_model/Subsystem1/MATLAB Function10 ==
  data: T input; Ax output; Ax_tr input; Ax_li input; Ax_s input; Ax_c input
function Ax = fcn(T,Ax_tr,Ax_li,Ax_s,Ax_c)
if T>=260 && T<=530
    Ax=Ax_tr
elseif T>=675 && T<=905
    Ax=Ax_s
elseif T>=1005 && T<=1285
    Ax=Ax_c
else
    Ax=Ax_li
end

== matlab function Inverse_model/Subsystem1/MATLAB Function1 ==
  data: T0 input; x_li output; T1 input; T4 input; T5 input; T7 input; T8 input; T9 input; T10 input; X0 input; X1 input; X4 input; X5 input; X7 input; X8 input; X9 input; X10 input; Y0 input; Y1 input; y_li output; Vx_li output; Vy_li output; Ax_li output; Ay_li output; t_li output; Y4 input; Y5 input; Y7 input; Y8 input; Y9 input; Y10 input
function [x_li,y_li,Vx_li,Vy_li,Ax_li,Ay_li,t_li] = fcn(T0,T1,T4,T5,T7,T8,T9,T10,X0,X1,X4,X5,X7,X8,X9,X10,Y0,Y1,Y4,Y5,Y7,Y8,Y9,Y10)
T0=0;
T1=260;
T4=530;
T5=675;
T7=905;
T8=1005;
T9=1285;
T10=1400;
X1=0.5;
X4=0.5;
X0=3;
Y0=2;
X5=1.75;
X7=1.75;
Y5=1.5;
Y7=1.5;
X8=2.75;
X9=2.75;
X10=3;
Y10=2;
Y8=1;
Y9=1;
Y1=0.5;
Y4=0.5;
sigma=0:0.01:1;
t0=T0+sigma*(T1-T0);
t4=T4+sigma*(T5-T4);
t7=T7+sigma*(T8-T7);
t9=T9+sigma*(T10-T9);
t_li=[t0 t4 t7 t9];
lambda=poly5(sigma);
x0=X0+lambda*(X1-X0);
x4=X4+lambda*(X5-X4);
x7=X7+lambda*(X8-X7);
x9=X9+lambda*(X10-X9);
x_li=[x0 x4 x7 x9];
y0=Y0+lambda*(Y1-Y0);
y4=Y4+lambda*(Y5-Y4);
y7=Y7+lambda*(Y8-Y7);
y9=Y9+lambda*(Y10-Y9);
y_li=[y0 y4 y7 y9];
lambdavel=poly5d(sigma);
Vx0=(X1-X0)/(T1-T0).*lambdavel;
Vx4=(X5-X4)/(T5-T4).*lambdavel;
Vx7=(X8-X7)/(T8-T7).*lambdavel;
Vx9=(X10-X9)/(T10-T9).*lambdavel;
Vy0=(Y1-Y0)/(T1-T0).*lambdavel;
Vy4=(Y5-Y4)/(T5-T4).*lambdavel;
Vy7=(Y8-Y7)/(T8-T7).*lambdavel;
Vy9=(Y10-Y9)/(T10-T9).*lambdavel;
lambdaac=poly5dd(sigma);
Ax0=(X1-X0)/(T1-T0)^2.*lambdaac;
Ax4=(X5-X4)/(T5-T4)^2.*lambdaac;
Ax7=(X8-X7)/(T8-T7)^2.*lambdaac;
Ax9=(X10-X9)/(T10-T9)^2.*lambdaac;
Ay0=(Y1-Y0)/(T1-T0)^2.*lambdaac;
Ay4=(Y5-Y4)/(T5-T4)^2.*lambdaac;
Ay7=(Y8-Y7)/(T8-T7)^2.*lambdaac;
Ay9=(Y10-Y9)/(T10-T9)^2.*lambdaac;
Vx_li=[Vx0 Vx4 Vx7 Vx9];
Vy_li=[Vy0 Vy4 Vy7 Vy9];
Ax_li=[Ax0 Ax4 Ax7 Ax9];
Ay_li=[Ay0 Ay4 Ay7 Ay9];

== matlab function Inverse_model/Subsystem1/MATLAB Function ==
  data: T1 input; x_tr output; T2 input; T3 input; T4 input; X1 input; X2 input; X3 input; Y1 input; Y2 input; Y3 input; y_tr output; Vx_tr output; Vy_tr output; Ax_tr output; Ay_tr output; t_tr output
function [x_tr,y_tr,Vx_tr,Vy_tr,Ax_tr,Ay_tr,t_tr] = fcn(T1,T2,T3,T4,X1,X2,X3,Y1,Y2,Y3)
T1=260;
T2=330;
T3=460;
T4=530;
X1=0.5;
X2=1.25;
X3=0.25;
Y1=0.5;
Y2=0.25;
Y3=1.25;
sigma=0:0.01:1;
t1=T1+sigma*(T2-T1);
t2=T2+sigma*(T3-T2);
t3=T3+sigma*(T4-T3);
t_tr=[t1 t2 t3];
lambda=poly5(sigma);
x1=X1+lambda*(X2-X1);
x2=X2+lambda*(X3-X2);
x3=X3+lambda*(X1-X3);
y1=Y1+lambda*(Y2-Y1);
y2=Y2+lambda*(Y3-Y2);
y3=Y3+lambda*(Y1-Y3);
lambdavel=poly5d(sigma);
Vx1=(X2-X1)/(T2-T1).*lambdavel;
Vx2=(X3-X2)/(T3-T2).*lambdavel;
Vx3=(X1-X3)/(T4-T3).*lambdavel;
Vy1=(Y2-Y1)/(T2-T1).*lambdavel;
Vy2=(Y3-Y2)/(T3-T2).*lambdavel;
Vy3=(Y1-Y3)/(T4-T3).*lambdavel; 
lambdaac=poly5dd(sigma);
Ax1=(X2-X1)/(T2-T1)^2.*lambdaac;
Ax2=(X3-X2)/(T3-T2)^2.*lambdaac;
Ax3=(X1-X3)/(T4-T3)^2.*lambdaac;
Ay1=(Y2-Y1)/(T2-T1)^2.*lambdaac;
Ay2=(Y3-Y2)/(T3-T2)^2.*lambdaac;
Ay3=(Y1-Y3)/(T4-T3)^2.*lambdaac; 

x_tr=[x1 x2 x3];
y_tr=[y1 y2 y3];
Vx_tr=[Vx1 Vx2 Vx3];
Vy_tr=[Vy1 Vy2 Vy3];
Ax_tr=[Ax1 Ax2 Ax3];
Ay_tr=[Ay1 Ay2 Ay3];

== matlab function Inverse_model/Subsystem1/MATLAB Function2 ==
  data: x_s output; T5 input; T6 input; T7 input; X6 input; Y6 input; X5 input; Y5 input; y_s output; Vx_s output; Vy_s output; Ax_s output; Ay_s output; t_s output
function [x_s,y_s,Vx_s,Vy_s,Ax_s,Ay_s,t_s] = fcn(T5,T6,T7,X6,Y6,X5,Y5)
T5=675;
T6=815;
T7=905;
X6=0.75;
X5=1.75;
Y6=1.5;
Y5=1.5;
t5=T5:0.1:T6;
sigm=(t5-T5)/(T6-T5);
lambda=poly5(sigm);
theta=lambda*pi;
R=0.5;
P=R*[cos(theta);sin(theta)];
x5=P(1,:)+1.25;
y5=P(2,:)+1.5;
lambdavelo=poly5d(sigm);
Vx5=R*[-sin(theta)]*2*pi/(T6-T5).*lambdavelo;
Vy5=R*[cos(theta)]*2*pi/(T6-T5).*lambdavelo;
lambdaacc=poly5dd(sigm);
Ax5=R*[-sin(theta)]*2*pi/(T6-T5)^2.*lambdaacc;
Ay5=R*[cos(theta)]*2*pi/(T6-T5)^2.*lambdaacc;
sigma=0:0.01:1;
t6=T6+sigma*(T7-T6);
lambda=poly5(sigma);
x6=X6+lambda*(X5-X6);
y6=Y6+lambda*(Y5-Y6);
lambdavel=poly5d(sigma);
lambdaac=poly5d(sigma);
Vx6=(X5-X6)/(T7-T6).*lambdavel;
Vy6=(Y5-Y6)/(T7-T6).*lambdavel;
Ax6=(X5-X6)/(T7-T6)^2.*lambdaac;
Ay6=(Y5-Y6)/(T7-T6)^2.*lambdaac;
x_s=[x5 x6];
y_s=[y5 y6];
Vx_s=[Vx5 Vx6];
Vy_s=[Vy5 Vy6];
Ax_s=[Ax5 Ax6];
Ay_s=[Ay5 Ay6];
t_s=[t5 t6];
